simulink model "V_f_Control"  (R2023a)
settings: Solver=VariableStepAuto  StartTime=0.0  StopTime=10  RelTol=1e-3
model workspace (MAT data in the model file):
  Vd = 835.155
libraries: sharedutil x6, aerolibutil x2, spsTriangleGeneratorLib x1, spspowerguiLib x1
settings Model: Creator=HP  LastModifiedBy=HP

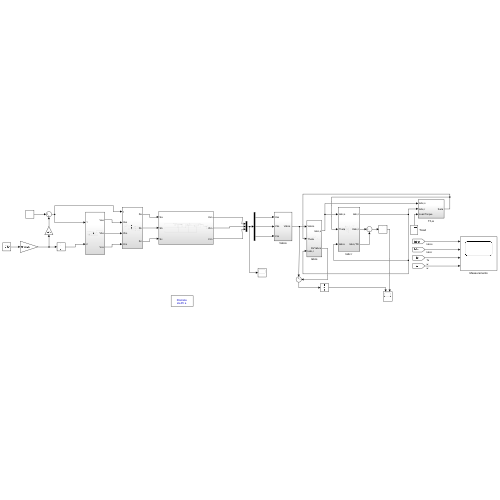
[thumbnail: Simulink's stored preview of the top-level diagram]
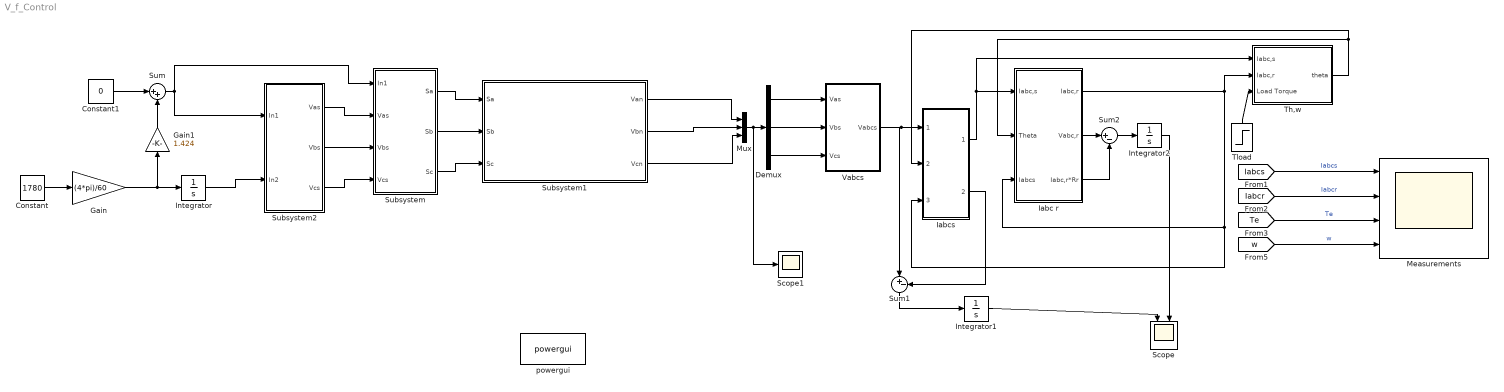
== system V_f_Control ==
  Constant : Constant  Value=1780
  Constant1 : Constant  Value=0
  Demux : Demux  Outputs=3
  Gain : Gain  Gain=(4*pi)/60
  Gain1 : Gain  Gain=1.424
  Iabc r : Subsystem
  Iabcs : Subsystem
  Integrator : Integrator
  Integrator1 : Integrator
  Integrator2 : Integrator
  "Measurements " : Scope  NumInputPorts=4
  Mux : Mux  Inputs=3
  Scope : Scope  NumInputPorts=2
  Scope1 : Scope
  Subsystem : Subsystem
  Subsystem1 : Subsystem
  Subsystem2 : Subsystem
  Sum : Sum  Inputs=|++
  Sum1 : Sum  Inputs=|+-
  Sum2 : Sum  Inputs=|+-
  Th,w : Subsystem
  Tload : Step  After=200  SampleTime=0
  Vabcs : Subsystem
  powergui : spspowerguiLib/powergui  Priority=1  SimulationMode=Discrete  SampleTime=20e-6  frequency=60  Iterations=50  frequencyindice=60  Pbase=100e6  ErrMax=1e-4  UnitsV=kV  UnitsW=MW  buscounter=0  FunctionMessages=off  echomessages=off  EnableUseOfTLC=off  CurrentSourceSwitches=off  DisableSnubberDevices=off  DisableRonSwitches=off  DisableVfSwitches=off  DisplayEquations=off  AutomaticDiscreteSolvers=off  SolverType=Tustin/Backward Euler (TBE)  Interpol=off  ExternalGateDelay=off  methode=off  Ts=100  x0status=blocks  SPID=on  SwTol=0  HookPort=off  NonlinearTolerance=1e-4  nMaxIteration=100  ContinueOnMaxIteration=off  RestoreLinks=warning  ResistiveCurrentMeasurement=off  Frange=[0:2:500]  Ylog=off  Xlog=on  ShowGrid=off  save=off  variable=ZData  structure=0  ZoomFFT=off  StartTime=0.0  cycles=1  DisplayStyle=1  fundamental=60  FreqAxis=off  MaxFrequency=1000  frequencyindicesteady=1  RmsSteady=1  display=off
  wires:
  Subsystem/1(Sa) -> Subsystem1/1(Sa)
  Subsystem/2(Sb) -> Subsystem1/2(Sb)
  Subsystem/3(Sc) -> Subsystem1/3(Sc)
  Gain/1 -> Integrator/1, Gain1/1
  Gain1/1 -> Sum/2
  Sum/1 -> Subsystem/1(In1), Subsystem2/1(In1)
  Integrator/1 -> Subsystem2/2(In2)
  Constant/1 -> Gain/1
  Constant1/1 -> Sum/1
  Subsystem2/1(Vas) -> Subsystem/2(Vas)
  Subsystem2/2(Vbs) -> Subsystem/3(Vbs)
  Subsystem2/3(Vcs) -> Subsystem/4(Vcs)
  Sum2/1 -> Integrator2/1
  Integrator2/1 -> Scope/2
  Integrator1/1 -> Scope/1
  Iabc r/2(Vabc,r) -> Sum2/1
  Tload/1 -> Th,w/3(Load Torque)
  Sum1/1 -> Integrator1/1
  Iabc r/3(Iabc,r*Rr) -> Sum2/2
  [Iabcs] -> "Measurements "/1  "Iabcs"
  Subsystem1/3(Vcn) -> Mux/3
  [Te] -> "Measurements "/3  "Te"
  Demux/2 -> Vabcs/2(Vbs)
  Vabcs/1("Vabcs ") -> Sum1/1, Iabcs/1(Vabcs)
  Th,w/1(theta) -> Iabcs/2(Theta), Iabc r/2(Theta)
  Iabcs/2(Rs*Iabcs) -> Sum1/2
  [Iabcr] -> "Measurements "/2  "Iabcr"
  Iabc r/1(Iabc,r) -> Th,w/2(Iabc,r), Iabcs/3(Iabc,r), Iabc r/3(Iabcs)
  [w] -> "Measurements "/4  "w"
  Demux/3 -> Vabcs/3(Vcs)
  Mux/1 -> Scope1/1, Demux/1
  Iabcs/1(Iabc,s) -> Iabc r/1(Iabc,s), Th,w/1(Iabc,s)
  Subsystem1/1(Van) -> Mux/1
  Demux/1 -> Vabcs/1(Vas)
  Subsystem1/2(Vbn) -> Mux/2

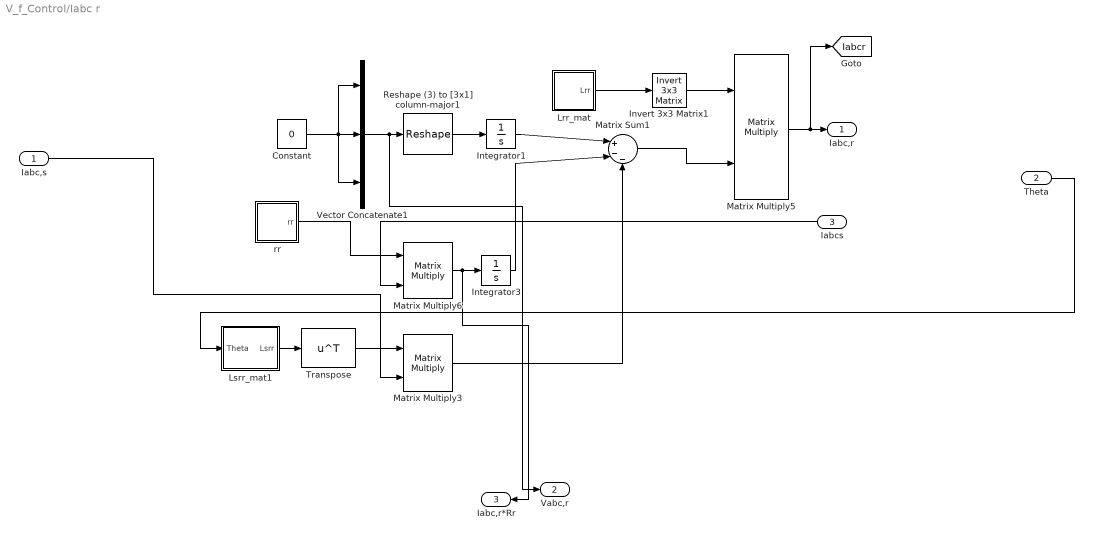
== system V_f_Control/Iabc r ==
  Iabc,s : Inport
  Theta : Inport  Port=2
  Iabcs : Inport  Port=3
  Constant : Constant  Value=0
  Integrator1 : Integrator
  Integrator3 : Integrator
  Invert 3x3 Matrix1 : aerolibutil/Invert  3x3 Matrix
  Lrr_mat : Subsystem
  Lsrr_mat1 : Subsystem
  Matrix Sum1 : Sum  Inputs=|+--
  Matrix Multiply3 : Product  Multiplication=Matrix(*)
  Matrix Multiply5 : Product  Multiplication=Matrix(*)
  Matrix Multiply6 : Product  Multiplication=Matrix(*)
  Reshape (3) to [3x1] column-major1 : Reshape  OutputDimensionality=Customize  OutputDimensions=[3,1]
  Transpose : Math  Operator=transpose
  Vector Concatenate1 : Concatenate  NumInputs=3
  rr : Subsystem
  Iabc,r : Outport
  Vabc,r : Outport  Port=2
  Iabc,r*Rr : Outport  Port=3
  tag scope: Iabcr=global
  wires:
  Matrix Multiply6/1 -> Iabc,r*Rr/1, Integrator3/1
  Integrator1/1 -> Matrix Sum1/1
  Theta/1 -> Lsrr_mat1/1(Theta)
  Iabc,s/1 -> Matrix Multiply3/2
  Constant/1 -> Vector Concatenate1/3, Vector Concatenate1/1, Vector Concatenate1/2
  Lrr_mat/1(Lrr) -> Invert 3x3 Matrix1/1
  Reshape (3) to [3x1] column-major1/1 -> Integrator1/1
  Vector Concatenate1/1 -> Vabc,r/1, Reshape (3) to [3x1] column-major1/1
  rr/1(rr) -> Matrix Multiply6/1
  Matrix Sum1/1 -> Matrix Multiply5/2
  Matrix Multiply3/1 -> Matrix Sum1/3
  Integrator3/1 -> Matrix Sum1/2
  Invert 3x3 Matrix1/1 -> Matrix Multiply5/1
  Matrix Multiply5/1 -> Iabc,r/1, [Iabcr]
  Iabcs/1 -> Matrix Multiply6/2
  Lsrr_mat1/1(Lsrr) -> Transpose/1
  Transpose/1 -> Matrix Multiply3/1

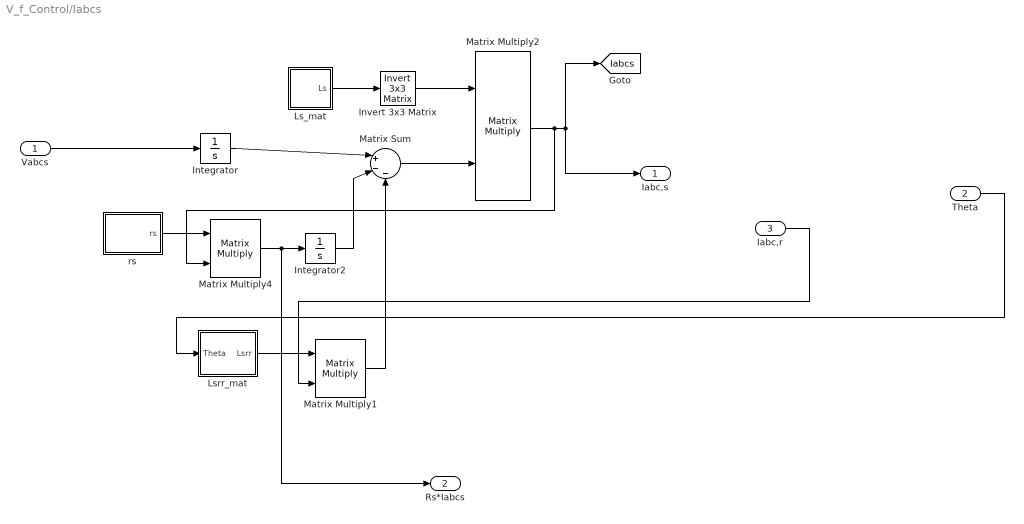
== system V_f_Control/Iabcs ==
  Vabcs : Inport
  Theta : Inport  Port=2
  Iabc,r : Inport  Port=3
  Integrator : Integrator
  Integrator2 : Integrator
  Invert 3x3 Matrix : aerolibutil/Invert  3x3 Matrix
  Ls_mat : Subsystem
  Lsrr_mat : Subsystem
  Matrix Sum : Sum  Inputs=|+--
  Matrix Multiply1 : Product  Multiplication=Matrix(*)
  Matrix Multiply2 : Product  Multiplication=Matrix(*)
  Matrix Multiply4 : Product  Multiplication=Matrix(*)
  rs : Subsystem
  Iabc,s : Outport
  Rs*Iabcs : Outport  Port=2
  tag scope: Iabcs=global
  wires:
  rs/1(rs) -> Matrix Multiply4/1
  Invert 3x3 Matrix/1 -> Matrix Multiply2/1
  Matrix Multiply4/1 -> Rs*Iabcs/1, Integrator2/1
  Vabcs/1 -> Integrator/1
  Ls_mat/1(Ls) -> Invert 3x3 Matrix/1
  Lsrr_mat/1(Lsrr) -> Matrix Multiply1/1
  Matrix Multiply2/1 -> Iabc,s/1, [Iabcs], Matrix Multiply4/2
  Matrix Multiply1/1 -> Matrix Sum/3
  Integrator2/1 -> Matrix Sum/2
  Matrix Sum/1 -> Matrix Multiply2/2
  Integrator/1 -> Matrix Sum/1
  Theta/1 -> Lsrr_mat/1(Theta)
  Iabc,r/1 -> Matrix Multiply1/2

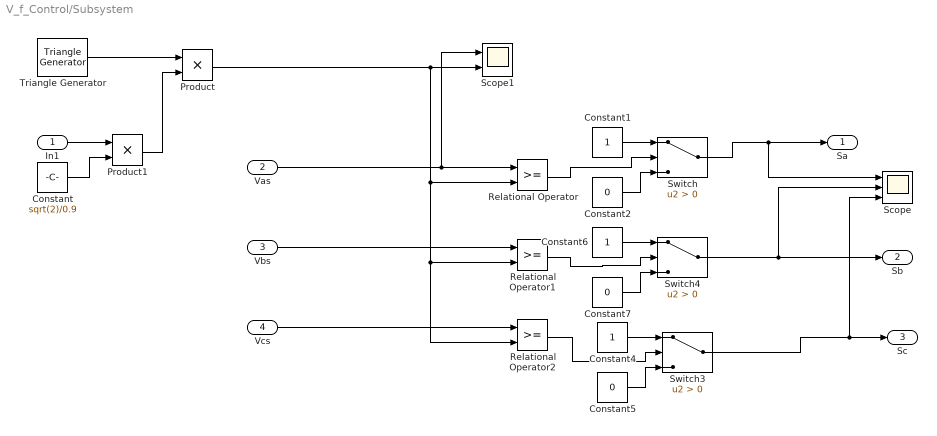
== system V_f_Control/Subsystem ==
  In1 : Inport
  Vas : Inport  Port=2
  Vbs : Inport  Port=3
  Vcs : Inport  Port=4
  Constant : Constant  Value=sqrt(2)/0.9
  Constant1 : Constant
  Constant2 : Constant  Value=0
  Constant4 : Constant
  Constant5 : Constant  Value=0
  Constant6 : Constant
  Constant7 : Constant  Value=0
  Product : Product
  Product1 : Product
  Relational Operator : RelationalOperator  OutDataTypeStr=boolean  RndMeth=Simplest  InputSameDT=off
  Relational Operator1 : RelationalOperator  OutDataTypeStr=boolean  RndMeth=Simplest  InputSameDT=off
  Relational Operator2 : RelationalOperator  OutDataTypeStr=boolean  RndMeth=Simplest  InputSameDT=off
  Scope : Scope  NumInputPorts=3
  Scope1 : Scope  NumInputPorts=2
  Switch : Switch  Criteria=u2 > Threshold  SaturateOnIntegerOverflow=off  InputSameDT=off
  Switch3 : Switch  Criteria=u2 > Threshold  SaturateOnIntegerOverflow=off  InputSameDT=off
  Switch4 : Switch  Criteria=u2 > Threshold  SaturateOnIntegerOverflow=off  InputSameDT=off
  Triangle Generator : spsTriangleGeneratorLib/Triangle Generator  Freq=40000  Phase=90  Ts=0
  Sa : Outport
  Sb : Outport  Port=2
  Sc : Outport  Port=3
  wires:
  Product/1 -> Scope1/2, Relational Operator2/2, Relational Operator1/2, Relational Operator/2
  Vcs/1 -> Relational Operator2/1
  Vbs/1 -> Relational Operator1/1
  Vas/1 -> Scope1/1, Relational Operator/1
  Triangle Generator/1 -> Product/1
  In1/1 -> Product1/1
  Constant/1 -> Product1/2
  Product1/1 -> Product/2
  Constant1/1 -> Switch/1
  Constant2/1 -> Switch/3
  Constant5/1 -> Switch3/3
  Constant4/1 -> Switch3/1
  Constant7/1 -> Switch4/3
  Constant6/1 -> Switch4/1
  Relational Operator/1 -> Switch/2
  Relational Operator1/1 -> Switch4/2
  Relational Operator2/1 -> Switch3/2
  Switch/1 -> Scope/1, Sa/1
  Switch4/1 -> Scope/2, Sb/1
  Switch3/1 -> Scope/3, Sc/1

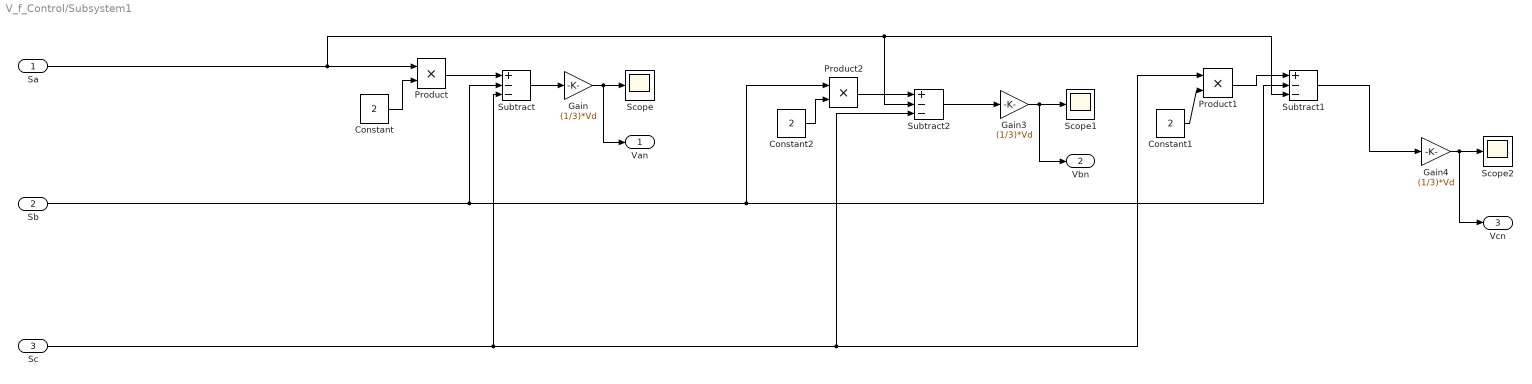
== system V_f_Control/Subsystem1 ==
  Sa : Inport
  Sb : Inport  Port=2
  Sc : Inport  Port=3
  Constant : Constant  Value=2
  Constant1 : Constant  Value=2
  Constant2 : Constant  Value=2
  Gain : Gain  Gain=(1/3)*Vd
  Gain3 : Gain  Gain=(1/3)*Vd
  Gain4 : Gain  Gain=(1/3)*Vd
  Product : Product
  Product1 : Product
  Product2 : Product
  Scope : Scope
  Scope1 : Scope
  Scope2 : Scope
  Subtract : Sum  Inputs=+--
  Subtract1 : Sum  Inputs=+--
  Subtract2 : Sum  Inputs=+--
  Van : Outport
  Vbn : Outport  Port=2
  Vcn : Outport  Port=3
  wires:
  Product/1 -> Subtract/1
  Sc/1 -> Product1/1, Subtract2/3, Subtract/3
  Product1/1 -> Subtract1/1
  Sa/1 -> Subtract2/2, Subtract1/3, Product/1
  Product2/1 -> Subtract2/1
  Sb/1 -> Subtract1/2, Product2/1, Subtract/2
  Constant2/1 -> Product2/2
  Subtract/1 -> Gain/1
  Constant/1 -> Product/2
  Gain3/1 -> Scope1/1, Vbn/1
  Subtract2/1 -> Gain3/1
  Gain4/1 -> Vcn/1, Scope2/1
  Subtract1/1 -> Gain4/1
  Gain/1 -> Van/1, Scope/1
  Constant1/1 -> Product1/2

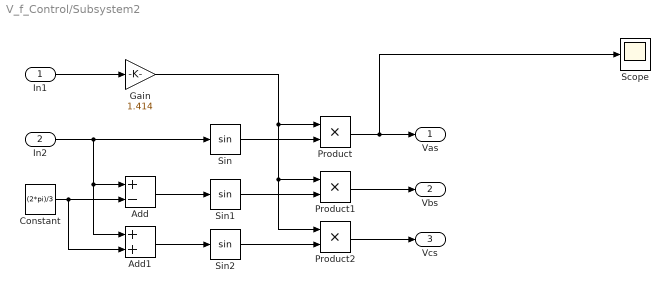
== system V_f_Control/Subsystem2 ==
  In1 : Inport
  In2 : Inport  Port=2
  Add : Sum  Inputs=+-
  Add1 : Sum
  Constant : Constant  Value=(2*pi)/3
  Gain : Gain  Gain=1.414
  Product : Product
  Product1 : Product
  Product2 : Product
  Scope : Scope
  Sin : Trigonometry
  Sin1 : Trigonometry
  Sin2 : Trigonometry
  Vas : Outport
  Vbs : Outport  Port=2
  Vcs : Outport  Port=3
  wires:
  In1/1 -> Gain/1
  In2/1 -> Add1/1, Add/1, Sin/1
  Constant/1 -> Add1/2, Add/2
  Add/1 -> Sin1/1
  Add1/1 -> Sin2/1
  Gain/1 -> Product2/1, Product1/1, Product/1
  Sin/1 -> Product/2
  Sin1/1 -> Product1/2
  Sin2/1 -> Product2/2
  Product/1 -> Scope/1, Vas/1
  Product1/1 -> Vbs/1
  Product2/1 -> Vcs/1

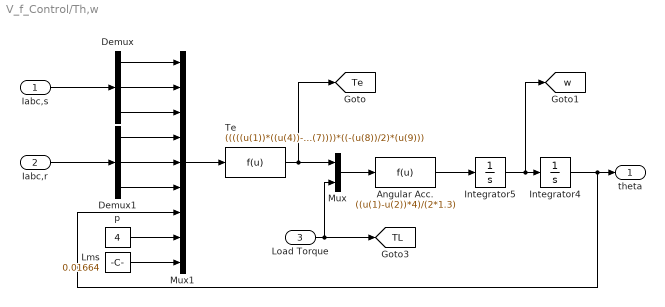
== system V_f_Control/Th,w ==
  Iabc,s : Inport
  Iabc,r : Inport  Port=2
  Load Torque : Inport  Port=3
  Angular Acc. : Fcn  Expr=((u(1)-u(2))*4)/(2*1.3)
  Demux : Demux  Outputs=3
  Demux1 : Demux  Outputs=3
  Integrator4 : Integrator
  Integrator5 : Integrator
  Lms : Constant  Value=0.01664
  Mux : Mux  Inputs=2
  Mux1 : Mux  Inputs=9
  Te : Fcn  Expr=(((((u(1))*((u(4))-(0.5*(u(5)))-(0.5*(u(6)))))+((u(2))*((u(5))-(0.5*(u(4)))-(0.5*(u(6)))))+((u(3))*((u(6))-(0.5*(u(5)))-(0.5*(u(4))))))*sin(u(7)))+((sqrt(3)/2)*(((u(1))*((u(5))-(u(6))))+((u(2))*((u(6))-(u(4))))+((u(3))*((u(4))-(u(5)))))*cos(u(7))))*((-(u(8))/2)*(u(9)))
  p : Constant  Value=4
  theta : Outport
  tag scope: TL=global, Te=global, w=global
  wires:
  Iabc,s/1 -> Demux/1
  Integrator4/1 -> Mux1/7, theta/1
  Mux/1 -> Angular Acc./1
  Load Torque/1 -> Mux/2, [TL]
  Angular Acc./1 -> Integrator5/1
  Te/1 -> [Te], Mux/1
  Integrator5/1 -> [w], Integrator4/1
  Iabc,r/1 -> Demux1/1
  Mux1/1 -> Te/1
  Demux/1 -> Mux1/1
  Demux/2 -> Mux1/2
  Demux/3 -> Mux1/3
  Demux1/1 -> Mux1/4
  Demux1/2 -> Mux1/5
  Demux1/3 -> Mux1/6
  p/1 -> Mux1/8
  Lms/1 -> Mux1/9

== system V_f_Control/Vabcs ==
  Vas : Inport
  Vbs : Inport  Port=2
  Vcs : Inport  Port=3
  Reshape (3) to [3x1] column-major : Reshape  OutputDimensionality=Customize  OutputDimensions=[3,1]
  Vector Concatenate : Concatenate  NumInputs=3
  "Vabcs " : Outport
  tag scope: Vabcs=global
  wires:
  Vector Concatenate/1 -> Reshape (3) to [3x1] column-major/1
  Reshape (3) to [3x1] column-major/1 -> [Vabcs], "Vabcs "/1
  Vbs/1 -> Vector Concatenate/2
  Vcs/1 -> Vector Concatenate/3
  Vas/1 -> Vector Concatenate/1

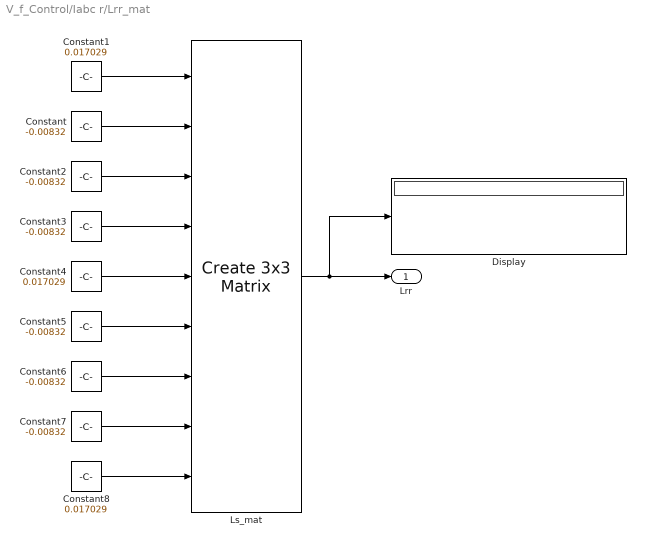
== system V_f_Control/Iabc r/Lrr_mat ==
  Constant{,2..3,5..7} (6 alike) : Constant  Value=-0.00832
  Constant1 : Constant  Value=0.017029
  Constant4 : Constant  Value=0.017029
  Constant8 : Constant  Value=0.017029
  Display : Display
  Ls_mat : sharedutil/Create 3x3 Matrix  aMode=aMode
      settings: LibrarySourceBlock=aerolibutil/Create 3x3 Matrix
  Lrr : Outport
  wires:
  Constant4/1 -> Ls_mat/5
  Constant5/1 -> Ls_mat/6
  Constant/1 -> Ls_mat/2
  Constant3/1 -> Ls_mat/4
  Constant1/1 -> Ls_mat/1
  Constant2/1 -> Ls_mat/3
  Constant6/1 -> Ls_mat/7
  Constant7/1 -> Ls_mat/8
  Constant8/1 -> Ls_mat/9
  Ls_mat/1 -> Display/1, Lrr/1

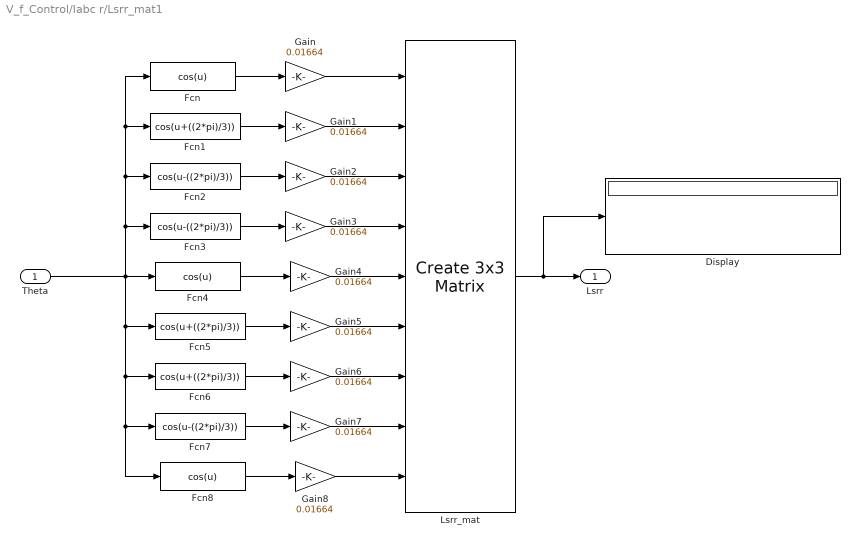
== system V_f_Control/Iabc r/Lsrr_mat1 ==
  Theta : Inport
  Display : Display
  Fcn : Fcn  Expr=cos(u)
  Fcn1 : Fcn  Expr=cos(u+((2*pi)/3))
  Fcn2 : Fcn  Expr=cos(u-((2*pi)/3))
  Fcn3 : Fcn  Expr=cos(u-((2*pi)/3))
  Fcn4 : Fcn  Expr=cos(u)
  Fcn5 : Fcn  Expr=cos(u+((2*pi)/3))
  Fcn6 : Fcn  Expr=cos(u+((2*pi)/3))
  Fcn7 : Fcn  Expr=cos(u-((2*pi)/3))
  Fcn8 : Fcn  Expr=cos(u)
  Gain{,1..8} (9 alike) : Gain  Gain=0.01664
  Lsrr_mat : sharedutil/Create 3x3 Matrix  aMode=aMode
      settings: LibrarySourceBlock=aerolibutil/Create 3x3 Matrix
  Lsrr : Outport
  wires:
  Fcn/1 -> Gain/1
  Fcn1/1 -> Gain1/1
  Fcn2/1 -> Gain2/1
  Gain/1 -> Lsrr_mat/1
  Gain1/1 -> Lsrr_mat/2
  Gain2/1 -> Lsrr_mat/3
  Fcn3/1 -> Gain3/1
  Gain3/1 -> Lsrr_mat/4
  Fcn4/1 -> Gain4/1
  Gain4/1 -> Lsrr_mat/5
  Fcn5/1 -> Gain5/1
  Gain5/1 -> Lsrr_mat/6
  Fcn6/1 -> Gain6/1
  Gain6/1 -> Lsrr_mat/7
  Fcn7/1 -> Gain7/1
  Gain7/1 -> Lsrr_mat/8
  Fcn8/1 -> Gain8/1
  Gain8/1 -> Lsrr_mat/9
  Theta/1 -> Fcn/1, Fcn1/1, Fcn2/1, Fcn3/1, Fcn5/1, Fcn6/1, Fcn8/1, Fcn7/1, Fcn4/1
  Lsrr_mat/1 -> Display/1, Lsrr/1

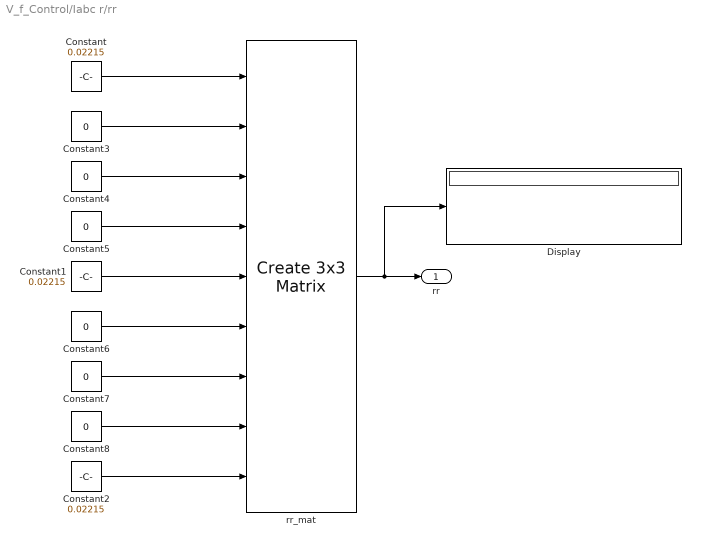
== system V_f_Control/Iabc r/rr ==
  Constant : Constant  Value=0.02215
  Constant1 : Constant  Value=0.02215
  Constant2 : Constant  Value=0.02215
  Constant{3..8} (6 alike) : Constant  Value=0
  Display : Display
  rr_mat : sharedutil/Create 3x3 Matrix  aMode=aMode
      settings: LibrarySourceBlock=aerolibutil/Create 3x3 Matrix
  rr : Outport
  wires:
  Constant/1 -> rr_mat/1
  Constant3/1 -> rr_mat/2
  Constant4/1 -> rr_mat/3
  Constant5/1 -> rr_mat/4
  Constant1/1 -> rr_mat/5
  Constant6/1 -> rr_mat/6
  Constant7/1 -> rr_mat/7
  Constant8/1 -> rr_mat/8
  Constant2/1 -> rr_mat/9
  rr_mat/1 -> Display/1, rr/1

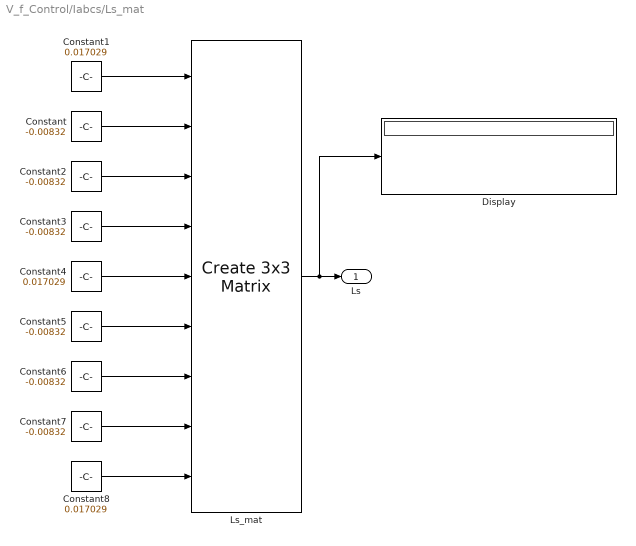
== system V_f_Control/Iabcs/Ls_mat ==
  Constant{,2..3,5..7} (6 alike) : Constant  Value=-0.00832
  Constant1 : Constant  Value=0.017029
  Constant4 : Constant  Value=0.017029
  Constant8 : Constant  Value=0.017029
  Display : Display
  Ls_mat : sharedutil/Create 3x3 Matrix  aMode=aMode
      settings: LibrarySourceBlock=aerolibutil/Create 3x3 Matrix
  Ls : Outport
  wires:
  Constant4/1 -> Ls_mat/5
  Constant5/1 -> Ls_mat/6
  Constant/1 -> Ls_mat/2
  Constant3/1 -> Ls_mat/4
  Constant1/1 -> Ls_mat/1
  Constant2/1 -> Ls_mat/3
  Constant6/1 -> Ls_mat/7
  Constant7/1 -> Ls_mat/8
  Constant8/1 -> Ls_mat/9
  Ls_mat/1 -> Display/1, Ls/1

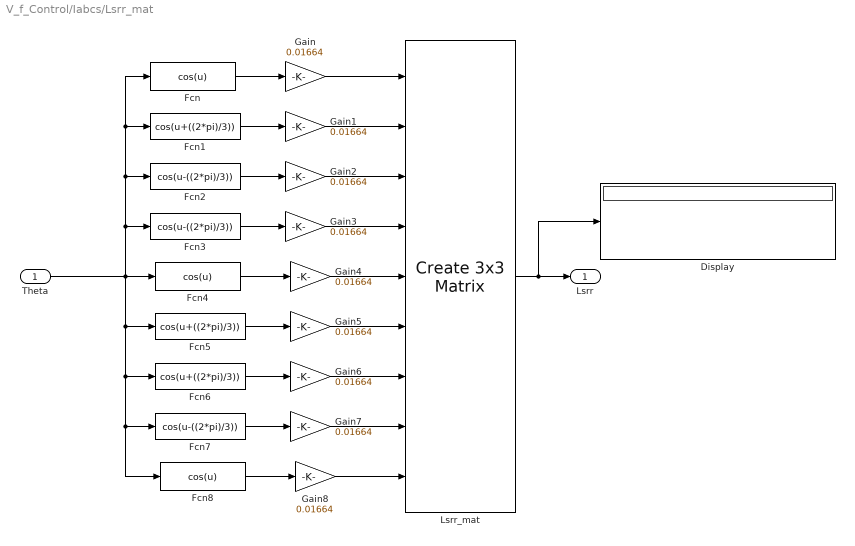
== system V_f_Control/Iabcs/Lsrr_mat ==
  Theta : Inport
  Display : Display
  Fcn : Fcn  Expr=cos(u)
  Fcn1 : Fcn  Expr=cos(u+((2*pi)/3))
  Fcn2 : Fcn  Expr=cos(u-((2*pi)/3))
  Fcn3 : Fcn  Expr=cos(u-((2*pi)/3))
  Fcn4 : Fcn  Expr=cos(u)
  Fcn5 : Fcn  Expr=cos(u+((2*pi)/3))
  Fcn6 : Fcn  Expr=cos(u+((2*pi)/3))
  Fcn7 : Fcn  Expr=cos(u-((2*pi)/3))
  Fcn8 : Fcn  Expr=cos(u)
  Gain{,1..8} (9 alike) : Gain  Gain=0.01664
  Lsrr_mat : sharedutil/Create 3x3 Matrix  aMode=aMode
      settings: LibrarySourceBlock=aerolibutil/Create 3x3 Matrix
  Lsrr : Outport
  wires:
  Fcn/1 -> Gain/1
  Fcn1/1 -> Gain1/1
  Fcn2/1 -> Gain2/1
  Gain/1 -> Lsrr_mat/1
  Gain1/1 -> Lsrr_mat/2
  Gain2/1 -> Lsrr_mat/3
  Fcn3/1 -> Gain3/1
  Gain3/1 -> Lsrr_mat/4
  Fcn4/1 -> Gain4/1
  Gain4/1 -> Lsrr_mat/5
  Fcn5/1 -> Gain5/1
  Gain5/1 -> Lsrr_mat/6
  Fcn6/1 -> Gain6/1
  Gain6/1 -> Lsrr_mat/7
  Fcn7/1 -> Gain7/1
  Gain7/1 -> Lsrr_mat/8
  Fcn8/1 -> Gain8/1
  Gain8/1 -> Lsrr_mat/9
  Theta/1 -> Fcn/1, Fcn1/1, Fcn2/1, Fcn3/1, Fcn5/1, Fcn6/1, Fcn8/1, Fcn7/1, Fcn4/1
  Lsrr_mat/1 -> Display/1, Lsrr/1

== system V_f_Control/Iabcs/rs ==
  Constant : Constant  Value=0.03957
  Constant1 : Constant  Value=0.03957
  Constant2 : Constant  Value=0.03957
  Constant{3..8} (6 alike) : Constant  Value=0
  Display : Display
  rs_mat : sharedutil/Create 3x3 Matrix  aMode=aMode
      settings: LibrarySourceBlock=aerolibutil/Create 3x3 Matrix
  rs : Outport
  wires:
  rs_mat/1 -> Display/1, rs/1
  Constant/1 -> rs_mat/1
  Constant3/1 -> rs_mat/2
  Constant4/1 -> rs_mat/3
  Constant5/1 -> rs_mat/4
  Constant1/1 -> rs_mat/5
  Constant6/1 -> rs_mat/6
  Constant7/1 -> rs_mat/7
  Constant8/1 -> rs_mat/8
  Constant2/1 -> rs_mat/9
